simulink library "Lib_Turbo_Valve_TMATS_new"  (R2015a)
settings: Solver=ode45  StartTime=0.0  StopTime=10.0  RelTol=1e-3
Description:
  | Thomas Modules
settings Model: Creator=jwchapm2  LastModifiedBy=jwhitfie
settings OptimizationCC: ExpressionDepthLimit=2147483647
settings DebuggingCC: UnderspecifiedInitializationDetection=Classic  MergeDetectMultiDrivingBlocksExec=none  SolverPrmCheckMsg=warning  StateNameClashWarn=warning

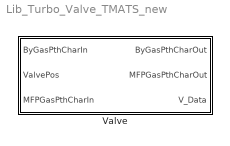
== system Lib_Turbo_Valve_TMATS_new ==
  Valve : Subsystem  mask(T-MATS: Valve Library Block){VFO_M=1, VDZ_M=0, VAe_M=20, X_VPRVec_M=[1 10], T_VWArray_M=[0 .99]}
      mask prompts: VFO_M "VFO_M - Valve fully open Value"; VDZ_M "VDZ_M - Valve dead zone Value"; VAe_M "VAe_M - Valve Active Area"; X_VPRVec_M "X_VPRVec_M - Valve Pressure Ratio Vector (x-axis)"; T_VWArray_M "T_VWArray_M - Valve Flow Array (W=f(PR))"
      mask help: This block simulates the performance of a valve using basic thermodynamic equations, properties, and table lookups.
      mask Help: web(which('Turbo_TMATS_Vlv.html'),'-helpbrowser')

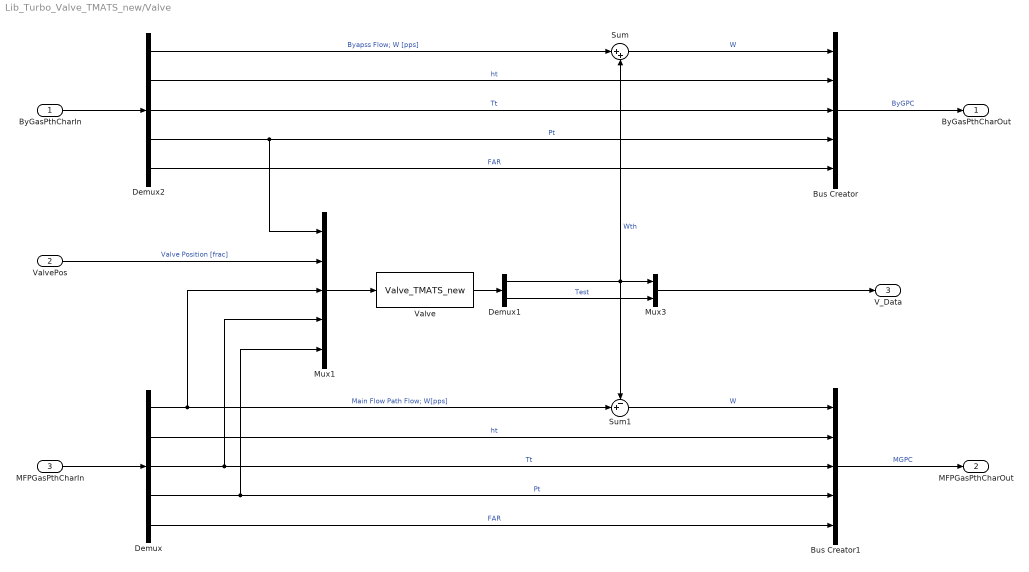
== system Lib_Turbo_Valve_TMATS_new/Valve ==
  ByGasPthCharIn : Inport
  ValvePos : Inport  Port=2
  MFPGasPthCharIn : Inport  Port=3
  Bus Creator : BusCreator  Inputs=5
  Bus Creator1 : BusCreator  Inputs=5
  Demux : Demux  Outputs=5
  Demux1 : Demux  Outputs=2
  Demux2 : Demux  Outputs=5
  Mux1 : Mux  Inputs=5
  Mux3 : Mux  Inputs=2
  Sum : Sum  Inputs=|++
  Sum1 : Sum  Inputs=-+|
  Valve : S-Function  FunctionName=Valve_TMATS_new  Parameters=VFO_M, VDZ_M, VAe_M, X_VPRVec_M, T_VWArray_M, gcs  SFunctionModules='interp1Ac_TMATS functions_TMATS'
  ByGasPthCharOut : Outport
  MFPGasPthCharOut : Outport  Port=2
  V_Data : Outport  Port=3
  wires:
  Bus Creator1/1 -> MFPGasPthCharOut/1  "MGPC"
  MFPGasPthCharIn/1 -> Demux/1
  Demux/5 -> Bus Creator1/5  "FAR"
  Demux/3 -> Mux1/4, Bus Creator1/3  "Tt"
  Demux/4 -> Bus Creator1/4, Mux1/5  "Pt"
  Mux1/1 -> Valve/1
  Demux/1 -> Sum1/2, Mux1/3  "Main Flow Path Flow; W[pps]"
  ValvePos/1 -> Mux1/2  "Valve Position [frac]"
  Demux1/1 -> Mux3/1, Sum1/1, Sum/2  "Wth"
  Valve/1 -> Demux1/1
  ByGasPthCharIn/1 -> Demux2/1
  Demux2/4 -> Mux1/1, Bus Creator/4  "Pt"
  Sum/1 -> Bus Creator/1  "W"
  Demux2/1 -> Sum/1  "Byapss Flow; W [pps]"
  Sum1/1 -> Bus Creator1/1  "W"
  Demux2/5 -> Bus Creator/5  "FAR"
  Demux2/3 -> Bus Creator/3  "Tt"
  Bus Creator/1 -> ByGasPthCharOut/1  "ByGPC"
  Demux1/2 -> Mux3/2  "Test"
  Mux3/1 -> V_Data/1
  Demux2/2 -> Bus Creator/2  "ht"
  Demux/2 -> Bus Creator1/2  "ht"
